simulink model "redundancy"  (R2023b)
settings: Solver=VariableStepAuto  StartTime=0.0  StopTime=10.0  RelTol=1e-3
settings Model: PauseTimes=0.1  Creator=Aniket  LastModifiedBy=Aniket
settings ConfigComp: DVTestSuiteOptimization=Auto  DVDetectOutOfBounds=on  DVModelReferenceHarness=on  DVHarnessSource=Signal Editor  DVRebuildModelRepresentation=IfChangeIsDetected

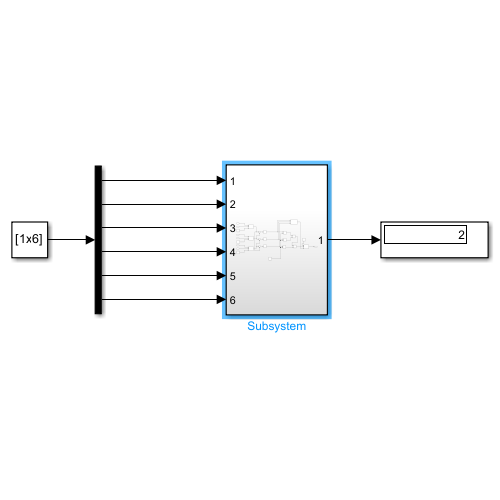
[thumbnail: Simulink's stored preview of the top-level diagram]
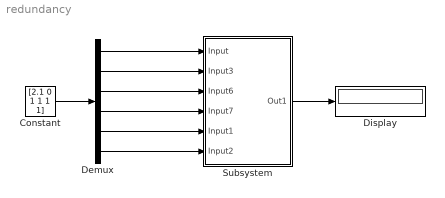
== system redundancy ==
  Constant : Constant  Value=[2.1 0 1 1 1 1]
  Demux : Demux  Outputs=6
  Display : Display
  Subsystem : Subsystem
  wires:
  Demux/1 -> Subsystem/1(Input)
  Demux/2 -> Subsystem/2(Input3)
  Demux/3 -> Subsystem/3(Input6)
  Demux/4 -> Subsystem/4(Input7)
  Demux/5 -> Subsystem/5(Input1)
  Demux/6 -> Subsystem/6(Input2)
  Subsystem/1(Out1) -> Display/1
  Constant/1 -> Demux/1

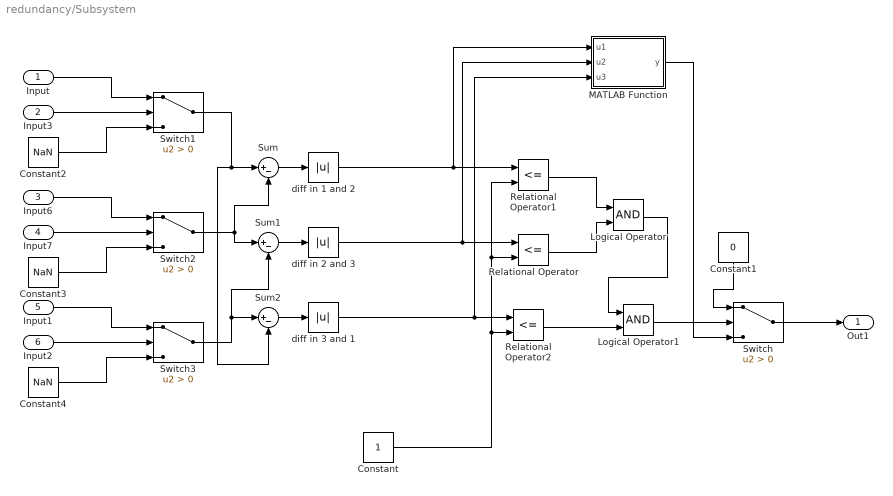
== system redundancy/Subsystem ==
  Input : Inport
  Input3 : Inport  Port=2
  Input6 : Inport  Port=3
  Input7 : Inport  Port=4
  Input1 : Inport  Port=5
  Input2 : Inport  Port=6
  Constant : Constant
  Constant1 : Constant  Value=0
  Constant2 : Constant  Value=NaN
  Constant3 : Constant  Value=NaN
  Constant4 : Constant  Value=NaN
  Logical Operator : Logic  AllPortsSameDT=off  OutDataTypeStr=boolean
  Logical Operator1 : Logic  AllPortsSameDT=off  OutDataTypeStr=boolean
  MATLAB Function : MATLAB Function  TreatAsAtomicUnit=on
  Relational Operator : RelationalOperator  Operator=<=  OutDataTypeStr=boolean  RndMeth=Simplest  InputSameDT=off
  Relational Operator1 : RelationalOperator  Operator=<=  OutDataTypeStr=boolean  RndMeth=Simplest  InputSameDT=off
  Relational Operator2 : RelationalOperator  Operator=<=  OutDataTypeStr=boolean  RndMeth=Simplest  InputSameDT=off
  Sum : Sum  Inputs=|+-
  Sum1 : Sum  Inputs=|+-
  Sum2 : Sum  Inputs=|+-
  Switch{,1..3} (4 alike) : Switch  Criteria=u2 > Threshold  SaturateOnIntegerOverflow=off  InputSameDT=off
  diff in 1 and 2 : Abs  SaturateOnIntegerOverflow=off
  diff in 2 and 3 : Abs  SaturateOnIntegerOverflow=off
  diff in 3 and 1 : Abs  SaturateOnIntegerOverflow=off
  Out1 : Outport
  wires:
  Relational Operator2/1 -> Logical Operator1/2
  Switch/1 -> Out1/1
  Input6/1 -> Switch2/1
  Sum1/1 -> diff in 2 and 3/1
  Relational Operator1/1 -> Logical Operator/1
  Switch2/1 -> Sum/2, Sum1/1
  Input3/1 -> Switch1/2
  Logical Operator1/1 -> Switch/2
  diff in 1 and 2/1 -> MATLAB Function/1(u1), Relational Operator1/1
  diff in 3 and 1/1 -> Relational Operator2/1, MATLAB Function/3(u3)
  Constant2/1 -> Switch1/3
  MATLAB Function/1(y) -> Switch/3
  diff in 2 and 3/1 -> Relational Operator/1, MATLAB Function/2(u2)
  Switch3/1 -> Sum1/2, Sum2/1
  Sum/1 -> diff in 1 and 2/1
  Constant/1 -> Relational Operator2/2, Relational Operator/2, Relational Operator1/2
  Switch1/1 -> Sum/1, Sum2/2
  Sum2/1 -> diff in 3 and 1/1
  Constant3/1 -> Switch2/3
  Input/1 -> Switch1/1
  Input7/1 -> Switch2/2
  Constant1/1 -> Switch/1
  Relational Operator/1 -> Logical Operator/2
  Logical Operator/1 -> Logical Operator1/1
  Constant4/1 -> Switch3/3
  Input1/1 -> Switch3/1
  Input2/1 -> Switch3/2

== matlab function redundancy/Subsystem/MATLAB Function ==
  data: u1 input; y output; u2 input; u3 input
function y = fcn(u1, u2, u3)
    if u1 < u2 && u1 < u3
        y = 3;
    elseif u2 < u1 && u2 < u3
        y = 1;
    else
        y = 2;
    end
end
